simulink model "sampleModel1421"  (R2023a)
settings: Solver=VariableStepAuto  StartTime=0.0  StopTime=10.0  RelTol=1e-3
libraries: simulink x6, hdlsllib x6
settings Model: Creator=user1  LastModifiedBy=user1

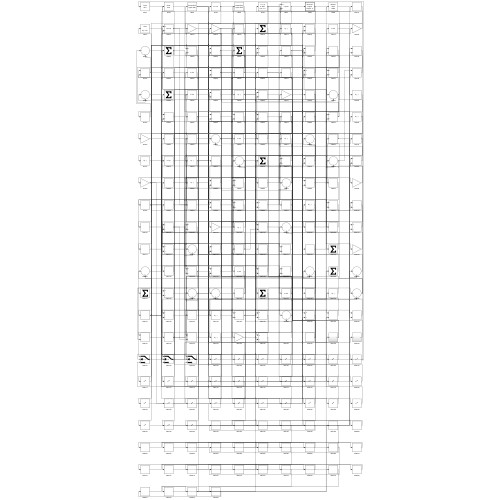
[thumbnail: Simulink's stored preview of the top-level diagram]
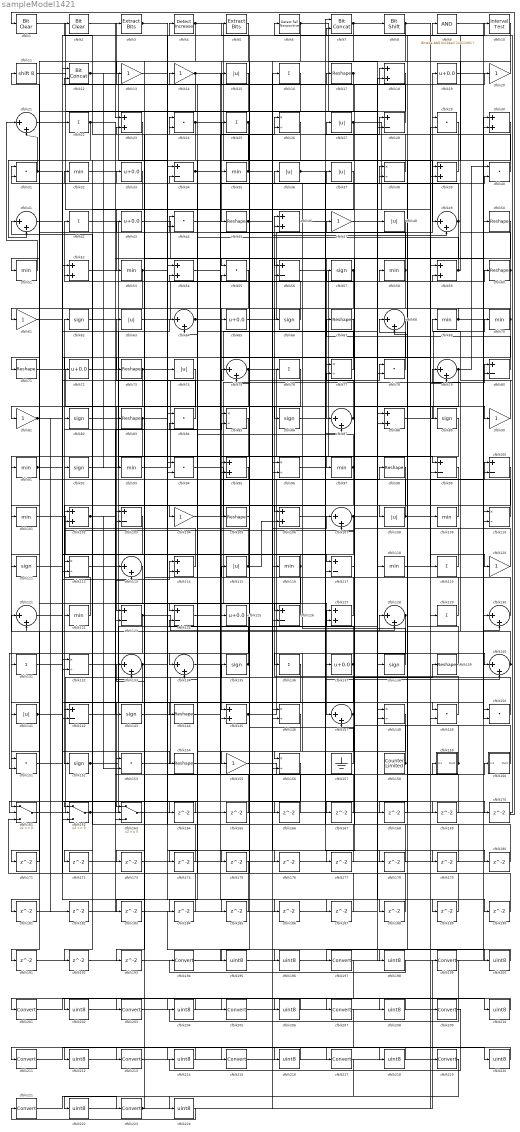
== system sampleModel1421 ==
  cfblk1 : simulink/Logic and Bit Operations/Bit Clear  iBit=0
      settings: LibrarySourceBlock=|
      | hdlsllib/Logic and Bit
      | Operations/Bit Clear
  cfblk10 : hdlsllib/Logic and Bit Operations/Interval Test  IntervalClosedRight=on  uplimit=0.5  IntervalClosedLeft=on  lowlimit=-0.5  OutDataTypeStr=boolean
  cfblk{28,34,56,80,99..100,103,117,123..124,126,142} (12 alike) : Sum  Inputs=+-
  cfblk{32,35,51,53,58,69..70,91,93,97,101,109,116,118,122} (15 alike) : MinMax
  cfblk{18,23,30,39,46,52,54,59,88,95,102,106,114,127,145} (15 alike) : Sum
  cfblk{13..14,20,47,61,81,90,104,120,155} (10 alike) : Gain
  cfblk{17,45,50,60,67,71,73,83,98,105,139,144,154} (13 alike) : Reshape
  cfblk{21,41,49,64,68,75,79,87,107,113,121,128,130,133..134,140,147} (17 alike) : Sum  Inputs=|++
  cfblk{15,27,36..37,48,63,74,108,115,141} (10 alike) : Abs  SaturateOnIntegerOverflow=off
  cfblk11 : ArithShift  BitShiftNumber=8
  cfblk{26,38,77,85,96,110,112,132,146,148,156} (11 alike) : Product  Inputs=*/  RndMeth=Zero  SaturateOnIntegerOverflow=on
  cfblk{57,62,66,82,86,89,92,111,135,138,143,152} (12 alike) : Signum
  cfblk{16,22,25,42,76,119,129,131,136} (9 alike) : Sum  Inputs=+
  cfblk12 : hdlsllib/Logic and Bit Operations/Bit Concat  numInputs=2
  cfblk{19,33,43,65,72,125,137} (7 alike) : Bias  Bias=0.0  SaturateOnIntegerOverflow=off
  cfblk{24,29,31,40,44,55,78,84,94,149..151,153} (13 alike) : DotProduct  OutDataTypeStr=Inherit: Inherit via internal rule
  cfblk157 : Ground
  cfblk158 : hdlsllib/Sources/Counter Limited  uplimit=7  tsamp=-1
  cfblk159 : Subsystem
      settings: LibrarySourceBlock=|
      | hdlsllib/Ports &
      | Subsystems/Subsystem
  cfblk160 : Subsystem
      settings: LibrarySourceBlock=|
      | hdlsllib/Ports &
      | Subsystems/Subsystem
  cfblk161 : Switch  SaturateOnIntegerOverflow=off  InputSameDT=off
  cfblk162 : Switch  SaturateOnIntegerOverflow=off  InputSameDT=off
  cfblk163 : Switch  SaturateOnIntegerOverflow=off  InputSameDT=off
  cfblk{164..193} (30 alike) : Delay  SampleTime=1
  cfblk{194,197,199,201,203,205,207,209,211,213,215,217,219,221,223} (15 alike) : DataTypeConversion  SaturateOnIntegerOverflow=off  RndMeth=Floor
  cfblk{195..196,198,200,202,204,206,208,210,212,214,216,218,220,222,224} (16 alike) : DataTypeConversion  OutDataTypeStr=uint8  SaturateOnIntegerOverflow=off  RndMeth=Floor
  cfblk2 : simulink/Logic and Bit Operations/Bit Clear  iBit=0
      settings: LibrarySourceBlock=|
      | hdlsllib/Logic and Bit
      | Operations/Bit Clear
  cfblk3 : simulink/Logic and Bit Operations/Extract Bits  bitsToExtract=Upper half  numBits=8  bitIdxRange=[0 7]  outScalingMode=Preserve fixed-point scaling
      settings: LibrarySourceBlock=|
      | hdlsllib/Logic and Bit
      | Operations/Extract Bits
  cfblk4 : simulink/Logic and Bit Operations/Detect Increase  vinit=0.0  OutDataTypeStr=boolean
      settings: LibrarySourceBlock=|
      | hdlsllib/Logic and Bit
      | Operations/Detect
      | Increase
  cfblk5 : simulink/Logic and Bit Operations/Extract Bits  bitsToExtract=Upper half  numBits=8  bitIdxRange=[0 7]  outScalingMode=Preserve fixed-point scaling
      settings: LibrarySourceBlock=|
      | hdlsllib/Logic and Bit
      | Operations/Extract Bits
  cfblk6 : hdlsllib/Logic and Bit Operations/Detect Fall Nonpositive  vinit=0  OutDataTypeStr=boolean
  cfblk7 : hdlsllib/Logic and Bit Operations/Bit Concat  numInputs=2
  cfblk8 : hdlsllib/Logic and Bit Operations/Bit Shift  mode=Shift Left Logical  N=0
  cfblk9 : simulink/Logic and Bit Operations/Bitwise Operator  logicop=AND  UseBitMask=on  BitMask=bin2dec('11011001')  BitMaskRealWorld=Stored Integer
      settings: LibrarySourceBlock=|
      | hdlsllib/Logic and Bit
      | Operations/Bitwise
      | Operator
  wires:
  cfblk79/1 -> cfblk40/1, cfblk177/1
  cfblk148/1 -> cfblk155/1
  cfblk42/1 -> cfblk97/1
  cfblk149/1 -> cfblk33/1
  cfblk122/1 -> cfblk62/1
  cfblk95/1 -> cfblk41/1
  cfblk139/1 -> cfblk6/1
  cfblk58/1 -> cfblk145/1, cfblk31/1, cfblk144/1
  cfblk60/1 -> cfblk61/1, cfblk100/2, cfblk7/2
  cfblk7/1 -> cfblk45/1, cfblk8/1
  cfblk147/1 -> cfblk46/1, cfblk175/1
  cfblk129/1 -> cfblk82/1
  cfblk44/1 -> cfblk26/1
  cfblk161/1 -> cfblk135/1
  cfblk70/1 -> cfblk65/1, cfblk126/2, cfblk156/2
  cfblk98/1 -> cfblk152/1
  cfblk12/1 -> cfblk74/1, cfblk93/1
  cfblk37/1 -> cfblk53/1
  cfblk134/1 -> cfblk40/2
  cfblk96/1 -> cfblk78/1
  cfblk137/1 -> cfblk147/2, cfblk56/2, cfblk24/2, cfblk192/1
  cfblk56/1 -> cfblk99/1
  cfblk154/1 -> cfblk46/2
  cfblk117/1 -> cfblk47/1
  cfblk32/1 -> cfblk55/1
  cfblk163/1 -> cfblk9/1
  cfblk48/1 -> cfblk87/1, cfblk73/1
  cfblk33/1 -> cfblk162/1
  cfblk107/1 -> cfblk140/1, cfblk173/1
  cfblk89/1 -> cfblk161/1
  cfblk78/1 -> cfblk68/1
  cfblk93/1 -> cfblk48/1
  cfblk22/1 -> cfblk41/2, cfblk133/2
  cfblk110/1 -> cfblk11/1
  cfblk26/1 -> cfblk134/1
  cfblk5/1 -> cfblk91/1
  cfblk85/1 -> cfblk141/1
  cfblk150/1 -> cfblk37/1
  cfblk62/1 -> cfblk145/2
  cfblk38/1 -> cfblk26/2
  cfblk65/1 -> cfblk19/1
  cfblk49/1 -> cfblk31/2, cfblk107/2, cfblk168/1
  cfblk66/1 -> cfblk42/1
  cfblk15/1 -> cfblk81/1
  cfblk74/1 -> cfblk123/1
  cfblk28/1 -> cfblk3/1
  cfblk39/1 -> cfblk35/1
  cfblk114/1 -> cfblk92/1
  cfblk130/1 -> cfblk27/1
  cfblk1/1 -> cfblk119/1
  cfblk4/1 -> cfblk49/1, cfblk183/1
  cfblk57/1 -> cfblk142/1, cfblk162/3
  cfblk64/1 -> cfblk117/1, cfblk38/1
  cfblk59/1 -> cfblk29/1, cfblk14/1
  cfblk27/1 -> cfblk109/1, cfblk83/1, cfblk189/1
  cfblk82/1 -> cfblk90/1
  cfblk51/1 -> cfblk21/1
  cfblk52/1 -> cfblk125/1
  cfblk116/1 -> cfblk112/1, cfblk172/1
  cfblk105/1 -> cfblk25/1
  cfblk88/1 -> cfblk70/1
  cfblk50/1 -> cfblk96/2
  cfblk23/1 -> cfblk122/1
  cfblk104/1 -> cfblk80/1
  cfblk111/1 -> cfblk75/1
  cfblk63/1 -> cfblk60/1
  cfblk90/1 -> cfblk69/1
  cfblk2/1 -> cfblk23/1
  cfblk84/1 -> cfblk63/1
  cfblk158/1 -> cfblk102/1, cfblk124/2
  cfblk138/1 -> cfblk36/1
  cfblk121/1 -> cfblk4/1
  cfblk119/1 -> cfblk34/2
  cfblk46/1 -> cfblk99/2
  cfblk20/1 -> cfblk13/1
  cfblk45/1 -> cfblk49/2, cfblk17/1
  cfblk47/1 -> cfblk20/1
  cfblk73/1 -> cfblk131/1, cfblk55/2, cfblk187/1
  cfblk80/1 -> cfblk67/1
  cfblk21/1 -> cfblk138/1
  cfblk131/1 -> cfblk114/1
  cfblk152/1 -> cfblk54/1, cfblk85/2
  cfblk162/1 -> cfblk139/1, cfblk160/1(In1)
  cfblk40/1 -> cfblk24/1
  cfblk36/1 -> cfblk28/1, cfblk140/2
  cfblk29/1 -> cfblk111/1
  cfblk157/1 -> cfblk5/1
  cfblk35/1 -> cfblk2/1, cfblk179/1
  cfblk94/1 -> cfblk147/1
  cfblk145/1 -> cfblk87/2, cfblk107/1
  cfblk72/1 -> cfblk137/1
  cfblk75/1 -> cfblk148/1, cfblk104/1, cfblk105/1
  cfblk31/1 -> cfblk52/1, cfblk21/2
  cfblk142/1 -> cfblk163/1
  cfblk143/1 -> cfblk16/1
  cfblk91/1 -> cfblk64/1, cfblk163/2
  cfblk81/1 -> cfblk117/2, cfblk181/1, cfblk182/1
  cfblk53/1 -> cfblk162/2, cfblk169/1
  cfblk133/1 -> cfblk153/1, cfblk10/1, cfblk150/2
  cfblk67/1 -> cfblk112/2
  cfblk68/1 -> cfblk103/2
  cfblk155/1 -> cfblk159/1(In1)
  cfblk97/1 -> cfblk64/2, cfblk134/2
  cfblk17/1 -> cfblk113/1, cfblk51/1
  cfblk83/1 -> cfblk190/1, cfblk191/1
  cfblk125/1 -> cfblk142/2
  cfblk159/1(Out1) -> cfblk127/1, cfblk57/1
  cfblk124/1 -> cfblk98/1
  cfblk14/1 -> cfblk151/1, cfblk56/1, cfblk101/1, cfblk86/1
  cfblk8/1 -> cfblk95/1, cfblk120/1
  cfblk9/1 -> cfblk150/1
  cfblk132/1 -> cfblk59/2
  cfblk43/1 -> cfblk110/2
  cfblk3/1 -> cfblk126/1, cfblk106/1, cfblk170/1
  cfblk10/1 -> cfblk39/1
  cfblk118/1 -> cfblk39/2
  cfblk141/1 -> cfblk22/1, cfblk154/1, cfblk149/1
  cfblk87/1 -> cfblk76/1, cfblk32/1
  cfblk34/1 -> cfblk89/1, cfblk79/2
  cfblk76/1 -> cfblk95/2
  cfblk135/1 -> cfblk115/1, cfblk54/2
  cfblk123/1 -> cfblk128/2, cfblk151/2
  cfblk25/1 -> cfblk123/2, cfblk72/1
  cfblk6/1 -> cfblk146/2, cfblk28/2, cfblk118/1, cfblk44/2
  cfblk86/1 -> cfblk7/1
  cfblk55/1 -> cfblk71/1
  cfblk92/1 -> cfblk58/1
  cfblk69/1 -> cfblk130/2, cfblk66/1
  cfblk160/1(Out1) -> cfblk15/1
  cfblk108/1 -> cfblk100/1, cfblk77/2
  cfblk128/1 -> cfblk121/2, cfblk136/1, cfblk156/1
  cfblk126/1 -> cfblk23/2
  cfblk112/1 -> cfblk113/2
  cfblk140/1 -> cfblk80/2, cfblk79/1, cfblk38/2
  cfblk11/1 -> cfblk88/1
  cfblk77/1 -> cfblk12/2
  cfblk61/1 -> cfblk18/1
  cfblk120/1 -> cfblk44/1
  cfblk109/1 -> cfblk108/1
  cfblk24/1 -> cfblk94/2, cfblk176/1
  cfblk153/1 -> cfblk129/1
  cfblk101/1 -> cfblk143/1
  cfblk115/1 -> cfblk84/2, cfblk106/2
  cfblk71/1 -> cfblk116/1
  cfblk19/1 -> cfblk50/1
  cfblk102/1 -> cfblk124/1, cfblk153/2
  cfblk127/1 -> cfblk102/2
  cfblk103/1 -> cfblk132/2
  cfblk146/1 -> cfblk164/1
  cfblk164/1 -> cfblk161/2
  cfblk54/1 -> cfblk165/1
  cfblk165/1 -> cfblk34/1
  cfblk41/1 -> cfblk166/1
  cfblk166/1 -> cfblk84/1
  cfblk100/1 -> cfblk167/1
  cfblk167/1 -> cfblk85/1
  cfblk168/1 -> cfblk68/2
  cfblk169/1 -> cfblk128/1
  cfblk170/1 -> cfblk1/1
  cfblk113/1 -> cfblk171/1
  cfblk171/1 -> cfblk121/1
  cfblk172/1 -> cfblk29/2
  cfblk173/1 -> cfblk130/1
  cfblk99/1 -> cfblk174/1
  cfblk174/1 -> cfblk94/1
  cfblk175/1 -> cfblk161/3
  cfblk176/1 -> cfblk18/2
  cfblk177/1 -> cfblk77/1
  cfblk106/1 -> cfblk178/1
  cfblk178/1 -> cfblk52/2
  cfblk179/1 -> cfblk127/2
  cfblk13/1 -> cfblk180/1
  cfblk180/1 -> cfblk133/1
  cfblk181/1 -> cfblk163/3
  cfblk182/1 -> cfblk78/2
  cfblk136/1 -> cfblk184/1
  cfblk184/1 -> cfblk132/1
  cfblk156/1 -> cfblk185/1
  cfblk185/1 -> cfblk12/1
  cfblk151/1 -> cfblk186/1
  cfblk186/1 -> cfblk148/2
  cfblk187/1 -> cfblk103/1
  cfblk144/1 -> cfblk188/1
  cfblk188/1 -> cfblk114/2
  cfblk189/1 -> cfblk75/2
  cfblk190/1 -> cfblk59/1
  cfblk191/1 -> cfblk88/2
  cfblk192/1 -> cfblk96/1
  cfblk16/1 -> cfblk193/1
  cfblk193/1 -> cfblk110/1
  cfblk18/1 -> cfblk195/1
  cfblk195/1 -> cfblk30/1
  cfblk183/1 -> cfblk196/1
  cfblk196/1 -> cfblk30/2
  cfblk30/1 -> cfblk198/1
  cfblk198/1 -> cfblk194/1
  cfblk194/1 -> cfblk200/1
  cfblk200/1 -> cfblk197/1
  cfblk197/1 -> cfblk202/1
  cfblk202/1 -> cfblk199/1
  cfblk199/1 -> cfblk204/1
  cfblk204/1 -> cfblk201/1
  cfblk201/1 -> cfblk206/1
  cfblk206/1 -> cfblk203/1
  cfblk203/1 -> cfblk208/1
  cfblk208/1 -> cfblk205/1
  cfblk205/1 -> cfblk210/1
  cfblk210/1 -> cfblk207/1
  cfblk207/1 -> cfblk212/1
  cfblk212/1 -> cfblk209/1
  cfblk209/1 -> cfblk214/1
  cfblk214/1 -> cfblk211/1
  cfblk211/1 -> cfblk216/1
  cfblk216/1 -> cfblk213/1
  cfblk213/1 -> cfblk218/1
  cfblk218/1 -> cfblk215/1
  cfblk215/1 -> cfblk220/1
  cfblk220/1 -> cfblk217/1
  cfblk221/1 -> cfblk223/1
  cfblk217/1 -> cfblk222/1
  cfblk222/1 -> cfblk219/1
  cfblk223/1 -> cfblk149/2, cfblk43/1, cfblk146/1
  cfblk219/1 -> cfblk224/1
  cfblk224/1 -> cfblk221/1

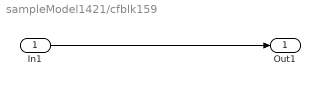
== system sampleModel1421/cfblk159 ==
  In1 : Inport
  Out1 : Outport
  wires:
  In1/1 -> Out1/1

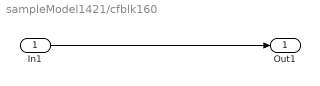
== system sampleModel1421/cfblk160 ==
  In1 : Inport
  Out1 : Outport
  wires:
  In1/1 -> Out1/1
